simulink model "SelfBalancingEV_V2"  (R2022a)
settings: Solver=VariableStepAuto  StartTime=0.0  StopTime=30  RelTol=1e-3
undefined symbols (not defined in the file): Ion, Lithium, sigbuilder_block, X, Y, Z
libraries: sm_lib x26, simulink x8, nesl_utility x6, fl_lib x3, slpidlib x2, spsControlledCurrentSourceLib x1, spsBatteryLib x1, spspowerguiLib x1
(part 1 of 2)
settings Model: Creator=DELL  LastModifiedBy=DELL
settings ConfigComp: CovScope=ReferencedModels

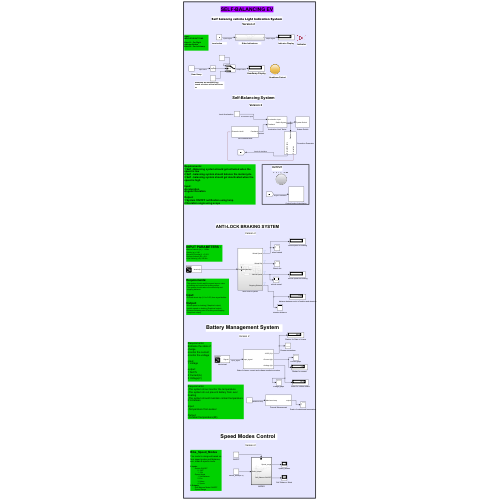
[thumbnail: Simulink's stored preview of the top-level diagram]
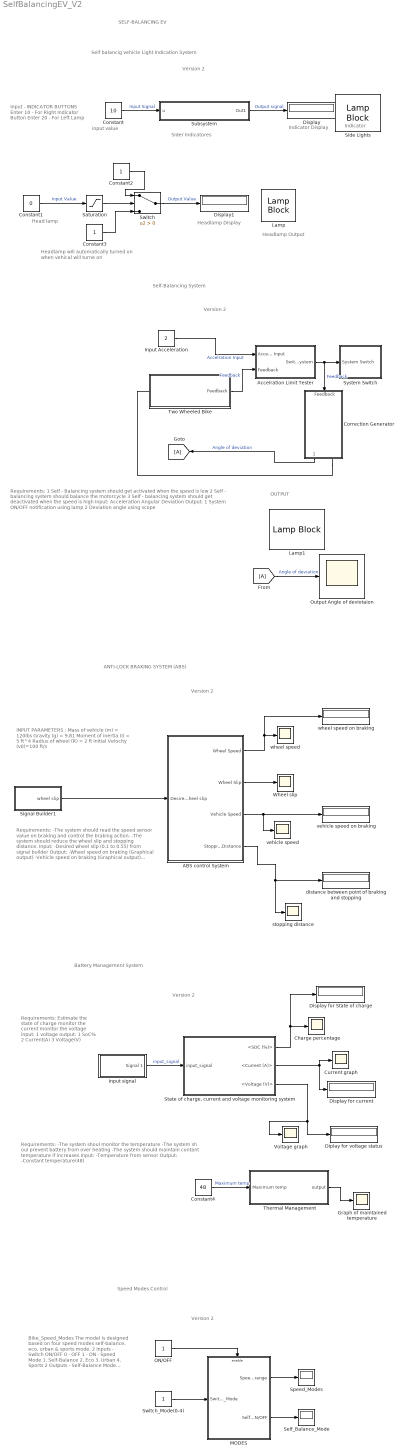
== system SelfBalancingEV_V2 ==
  note: SELF-BALANCING EV
  note: input value
  note: Head lamp
  note: Indicator Display
  note: Input -
      | INDICATOR BUTTONS
      |
      | Enter 10 - For Right Indicator Button
      | Enter 20 - For Left Lamp
  note: Indicator
  note: Version 2
  note: Headlamp Display
  note: Self balancig vehicle Light Indication System
  note: Headlamp will automatically turned on when vehical will turne on
  note: Sider Indicatores
  note: Headlamp Output
  note: Requirements:
      | -The system should read the speed sensor value
      | on braking and control the braking action.
      | -The system should reduce the wheel slip and
      | stopping distance.
      |
      | Input:
      | -Desired wheel slip (0.1 to 0.55) from signal builder
      |
      | Output:
      | -Wheel speed on braking (Graphical output)
      | -Vehicle speed on braking (Graphical output)
      | -Distance between point of braking and stopping
      | (Graphical output)
  note: INPUT PARAMETERS :
      | Mass of vehicle (m) = 120lbs
      | Gravity (g) = 9.81
      | Moment of inertia (I) = 5 ft^4
      | Radius of wheel (R) = 2 ft
      | Initial Velocity (v0)=100 ft/s
  note: ANTI-LOCK BRAKING SYSTEM (ABS)
  note: Version 2
  note: Requirements:
      | -The system shoul monitor the temperature
      | -The system sh oul prevent battery from over
      | heating
      | -The system should maintain contant temperature
      | if increases
      |
      | Input:
      | -Temperature from sensor
      |
      | Output:
      | -Constant temperature(48)
  note: Battery Management System
  note: Requirements:
      | Estimate the state of
      | charge
      | monitor the current
      | monitor the voltage
      |
      | input:
      | 1 voltage
      |
      | output:
      | 1 SoC%
      | 2 Current(A)
      | 3 Voltage(V)
  note: Bike_Speed_Modes
      |
      | The model is designed based on
      | four speed modes self-balance,
      | eco, urban & sports mode.
      |
      | 2 Inputs
      | - Switch ON/OFF
      | 0 - OFF
      | 1 - ON
      | - Speed Mode
      | 1. Self-Balance
      | 2. Eco
      | 3. Urban
      | 4. Sports
      | 2 Outputs
      | - Self-Balance Mode ON/OFF
      | - Speed Range
  note: Version 2
  note: Speed Modes Control
  note: Version 2
  note: Requirements:
      | 1 Self - Balancing system should get activated when the speed is low
      | 2 Self - balancing system should balance the motorcycle
      | 3 Self - balancing system should get deactivated when the speed is high
      |
      | Input:
      | Acceleration
      | Angular Deviation
      |
      | Output:
      | 1 System ON/OFF notification using lamp
      | 2 Deviation angle using scope
  note: Self-Balancing System
  note: OUTPUT
  note: Version 2
  ABS control System : Subsystem
  Accelration Limit Tester : Subsystem
  Charge percentage : Scope
  Constant : Constant  Value=10
  Constant1 : Constant  Value=0
  Constant2 : Constant
  Constant3 : Constant
  Constant4 : Constant  Value=48
  Correction Generator : Subsystem
  Current graph : Scope
  Diplay for voltage status : Display
  Display : Display
  Display for State of charge : Display
  Display for current : Display
  Display1 : Display
  From : From
  Goto : Goto
  Graph of maintained temperature : Scope
  Input Acceleration : Constant  Value=2
  Input signal : Subsystem  Tag=STV Subsys  LoadFcn=sigbuilder_block('load');  StartFcn=sigbuilder_block('start');  StopFcn=sigbuilder_block('stop');  ClipboardFcn=sigbuilder_block('clipboard');  mask(Sigbuilder block){tuvar=[0:10]}
      mask help: Simulink:masks:SigbuilderBlock_MD
      mask init:
      | if ~strcmp(get_param(bdroot(gcbh),'SimulationStatus'),'stopped') tuvar = sigbuilder_block('maskInit'); end
      settings: CopyFcn=sigbuilder_block('copy');  DeleteFcn=sigbuilder_block('delete');  ModelCloseFcn=sigbuilder_block('modelClose');  PreSaveFcn=sigbuilder_block('preSave');  PauseFcn=sigbuilder_block('pause');  ContinueFcn=sigbuilder_block('continue');  NameChangeFcn=sigbuilder_block('namechange');  OpenFcn=sigbuilder_block('open',[406.8 120.6 550.8 400.2 ]);  CloseFcn=sigbuilder_block('close');
      mask Display: plot(0, 0, 100, 100,[2, 2, 32, 32, 2], [68, 8, 8, 68, 68],[32, 2], [38, 38], [32, 19, 2],[53, 60, 44], [32, 17, 17, 2],[16, 16, 31, 31]);txt = getActiveGroup(gcbh);text(2, 100, txt,'verticalAlignment', 'top');
  Lamp : LampBlock  LabelPosition=Hide
  Lamp1 : LampBlock
  MODES : Subsystem
  ON/OFF : Constant
  "Output Angle of deviotaion " : Scope
  Saturation : Saturate  UpperLimit=1  LowerLimit=0
  Self_Balance_Mode : Display
  Side Lights : LampBlock  LabelPosition=Hide  Icon=SideLights
  Signal Builder1 : Subsystem  Tag=STV Subsys  LoadFcn=sigbuilder_block('load');  StartFcn=sigbuilder_block('start');  StopFcn=sigbuilder_block('stop');  ClipboardFcn=sigbuilder_block('clipboard');  mask(Sigbuilder block){tuvar=[0:10]}
      mask help: Simulink:masks:SigbuilderBlock_MD
      mask init:
      | if ~strcmp(get_param(bdroot(gcbh),'SimulationStatus'),'stopped') tuvar = sigbuilder_block('maskInit'); end
      settings: CopyFcn=sigbuilder_block('copy');  DeleteFcn=sigbuilder_block('delete');  ModelCloseFcn=sigbuilder_block('modelClose');  PreSaveFcn=sigbuilder_block('preSave');  PauseFcn=sigbuilder_block('pause');  ContinueFcn=sigbuilder_block('continue');  NameChangeFcn=sigbuilder_block('namechange');  OpenFcn=sigbuilder_block('open',[437.6 199.2 550.4 400 ]);  CloseFcn=sigbuilder_block('close');
      mask Display: plot(0, 0, 100, 100,[2, 2, 32, 32, 2], [68, 8, 8, 68, 68],[32, 2], [38, 38], [32, 19, 2],[53, 60, 44], [32, 17, 17, 2],[16, 16, 31, 31]);txt = getActiveGroup(gcbh);text(2, 100, txt,'verticalAlignment', 'top');
  Speed_Modes : Display
  "State of charge, current and voltage monitoring system" : Subsystem
  Subsystem : Subsystem
  Switch : Switch  Criteria=u2 > Threshold  SaturateOnIntegerOverflow=off  InputSameDT=off
  Switch_Mode(0-4) : Constant
  System Switch : Subsystem
  Thermal Management : Subsystem
  Two Wheeled Bike : Subsystem
  "Voltage graph " : Scope
  Wheel slip : Scope
  distance between point of braking and stopping : Display
  stopping distance : Scope
  vehicle speed : Scope
  vehicle speed on braking : Display
  wheel speed : Scope
  wheel speed on braking : Display
  wires:
  Constant1/1 -> Saturation/1  "Input Value"
  Subsystem/1(Out1) -> Display/1  "Output signal"
  Saturation/1 -> Switch/2
  Switch/1 -> Display1/1  "Output Value"
  Constant/1 -> Subsystem/1(u)  "Input Signal"
  Constant2/1 -> Switch/1
  Constant3/1 -> Switch/3
  ABS control System/4(Stopping Distance) -> distance between point of braking and stopping/1, stopping distance/1
  ABS control System/1(Wheel Speed) -> wheel speed/1, wheel speed on braking/1
  ABS control System/2(Wheel Slip) -> Wheel slip/1
  ABS control System/3(Vehicle Speed) -> vehicle speed on braking/1, vehicle speed/1
  Signal Builder1/1(wheel slip) -> ABS control System/1(Desired wheel slip)
  Constant4/1 -> Thermal Management/1(Maximum temp)  "Maximum temp"
  Input signal/1(Signal 1) -> "State of charge, current and voltage monitoring system"/1(input_signal)  "input_signal"
  "State of charge, current and voltage monitoring system"/1(<SOC (%)>) -> Display for State of charge/1, Charge percentage/1
  Thermal Management/1(output) -> Graph of maintained temperature/1
  "State of charge, current and voltage monitoring system"/2(<Current (A)>) -> Current graph/1, Display for current/1
  "State of charge, current and voltage monitoring system"/3(<Voltage (V)>) -> Diplay for voltage status/1, "Voltage graph "/1
  MODES/1(Speed_range) -> Speed_Modes/1
  MODES/2(Self_Balance ON/OFF) -> Self_Balance_Mode/1
  Switch_Mode(0-4)/1 -> MODES/1(Swithc_Mode)
  ON/OFF/1 -> MODES/Enable
  From/1 -> "Output Angle of deviotaion "/1  "Angle of deviation"
  Correction Generator/1(Deviation Angle) -> Goto/1  "Angle of deviation"
  Input Acceleration/1 -> Accelration Limit Tester/1(Acceleration Input)  "Accelration Input"
  Two Wheeled Bike/1(Feedback) -> Accelration Limit Tester/2("Feedback ")  "Feedback"
  Accelration Limit Tester/1(Switch System) -> System Switch/1(System Switch), Correction Generator/1(Feedback)  "Feedback"
  connections:
  Correction Generator/RConn1 -- Two Wheeled Bike/LConn1

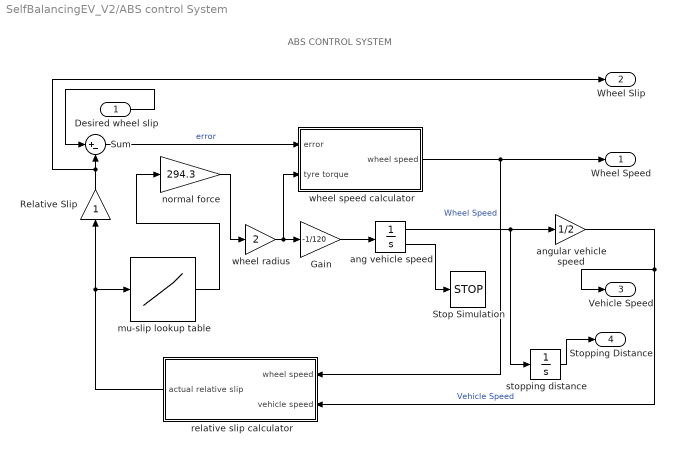
== system SelfBalancingEV_V2/ABS control System ==
  note: ABS CONTROL SYSTEM
  Desired wheel slip : Inport
  Gain : Gain  Gain=-1/120
  Relative Slip : Gain
  Stop Simulation : Stop
  Sum : Sum  Inputs=|+-
  ang vehicle speed : Integrator  InitialCondition=100  LimitOutput=on  UpperSaturationLimit=1000  LowerSaturationLimit=0  ShowSaturationPort=on
  angular vehicle speed : Gain  Gain=1/2
  mu-slip lookup table : Lookup_n-D  NumberOfTableDimensions=1  BreakpointsForDimension1=[0;0.05;0.1;0.15;0.2;0.25;0.3;0.35;0.4;0.45;0.5;0.55;0.6;0.65;0.7;0.75;0.8;0.85;0.9;0.95;1]  Table=[0;0.4;0.8;0.97;1;0.98;0.96;0.94;0.92;0.9;0.88;0.855;0.83;0.81;0.79;0.77;0.75;0.73;0.72;0.71;0.7]  InternalRulePriority=Speed  RndMeth=Simplest
  normal force : Gain  Gain=294.3
  relative slip calculator : Subsystem
  stopping distance : Integrator
  wheel radius : Gain  Gain=2
  wheel speed calculator : Subsystem
  Wheel Speed : Outport
  Wheel Slip : Outport  Port=2
  Vehicle Speed : Outport  Port=3
  Stopping Distance : Outport  Port=4
  wires:
  ang vehicle speed/1 -> angular vehicle speed/1, stopping distance/1
  relative slip calculator/1(actual relative slip) -> Relative Slip/1, mu-slip lookup table/1
  normal force/1 -> wheel radius/1
  wheel speed calculator/1(wheel speed) -> Wheel Speed/1, relative slip calculator/1(wheel speed)  "Wheel Speed"
  Sum/1 -> wheel speed calculator/1(error)  "error"
  angular vehicle speed/1 -> Vehicle Speed/1, relative slip calculator/2(vehicle speed)  "Vehicle Speed"
  Gain/1 -> ang vehicle speed/1
  wheel radius/1 -> Gain/1, wheel speed calculator/2(tyre torque)
  ang vehicle speed/2 -> Stop Simulation/1
  Relative Slip/1 -> Wheel Slip/1, Sum/2
  mu-slip lookup table/1 -> normal force/1
  stopping distance/1 -> Stopping Distance/1
  Desired wheel slip/1 -> Sum/1

== system SelfBalancingEV_V2/Accelration Limit Tester ==
  note: Requirement
      | 1 Acceleration tester which enables the system at low speed
      |
      | Input
      | 1 Acceleration
      |
      | Output
      | 1 Feedback
  note: Accelration Limit Tester
  Acceleration Input : Inport
  "Feedback " : Inport  Port=2
  Switch1 : Switch  Threshold=4  SaturateOnIntegerOverflow=off  InputSameDT=off
  const : Constant  Value=0
  Switch System : Outport
  wires:
  Acceleration Input/1 -> Switch1/2  "Acceleration Input"
  const/1 -> Switch1/1
  "Feedback "/1 -> Switch1/3  "Feedback"
  Switch1/1 -> Switch System/1  "Feedback"

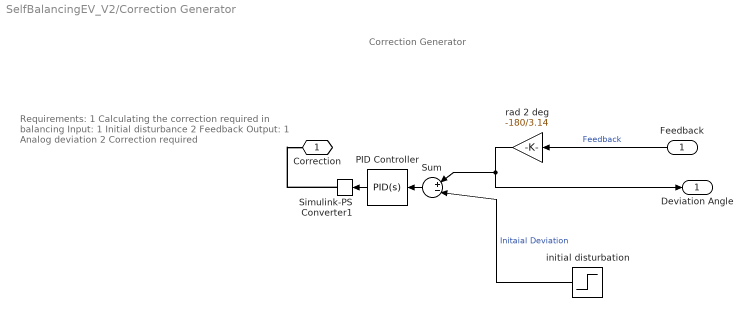
== system SelfBalancingEV_V2/Correction Generator ==
  note: Requirements:
      | 1 Calculating the correction required in balancing
      | Input:
      | 1 Initial disturbance
      | 2 Feedback
      |
      | Output:
      | 1 Analog deviation
      | 2 Correction required
  note: Correction Generator
  Feedback : Inport
  PID Controller : slpidlib/PID Controller  Controller=PID  Form=Parallel  TimeDomain=Continuous-time  UseExternalTs=off  SampleTime=-1  IntegratorMethod=Forward Euler  FilterMethod=Forward Euler  ControllerParametersSource=internal  P=2  I=5  UseKiTs=off  D=0.01  N=100  UseFilter=on  TunerSelectOption=Transfer Function Based (PID Tuner App)  InitialConditionSource=internal  InitialConditionForIntegrator=0  InitialConditionForFilter=0  DifferentiatorICPrevScaledInput=0  ExternalReset=none  TrackingMode=off  Kt=1  LimitOutput=off  SatLimitsSource=internal  UpperSaturationLimit=inf  LowerSaturationLimit=-inf  LinearizeAsGain=on  AntiWindupMode=none  Kb=1  POutMin=[]  POutMax=[]  IOutMin=[]  IOutMax=[]  DOutMin=[]  DOutMax=[]  NOutMin=[]  NOutMax=[]  SumOutMin=[]  SumOutMax=[]  SaturationOutMin=[]  SaturationOutMax=[]  PParamMin=[]  PParamMax=[]  IParamMin=[]  IParamMax=[]  DParamMin=[]  DParamMax=[]  NParamMin=[]  NParamMax=[]  KbParamMin=[]  KbParamMax=[]  KtParamMin=[]  KtParamMax=[]  KbOutMin=[]  KbOutMax=[]  KtOutMin=[]  KtOutMax=[]  IntegratorOutMin=[]  IntegratorOutMax=[]  FilterOutMin=[]  FilterOutMax=[]  SumI1OutMin=[]  SumI1OutMax=[]  SumI2OutMin=[]  SumI2OutMax=[]  SumI3OutMin=[]  SumI3OutMax=[]  SumI4OutMin=[]  SumI4OutMax=[]  SumDOutMin=[]  SumDOutMax=[]  DifferentiatorOutMin=[]  DifferentiatorOutMax=[]  FilterDiffOutCoefMin=[]  FilterDiffOutCoefMax=[]  ReciprocalOutMin=[]  ReciprocalOutMax=[]  SumDenOutMin=[]  SumDenOutMax=[]  SumNumOutMin=[]  SumNumOutMax=[]  DivideOutMin=[]  DivideOutMax=[]  UdiffTsProdOutMin=[]  UdiffTsProdOutMax=[]  NTsProdOutMin=[]  NTsProdOutMax=[]  UintegralTsProdOutMin=[]  UintegralTsProdOutMax=[]  UngainTsProdOutMin=[]  UngainTsProdOutMax=[]  IntegratorContinuousStateAttributes=''  IntegratorStateMustResolveToSignalObject=off  IntegratorRTWStateStorageClass=Auto  FilterContinuousStateAttributes=''  FilterStateMustResolveToSignalObject=off  FilterRTWStateStorageClass=Auto  ParallelPVariant=InternalParameters  IdealPVariant=Disabled  IVariant=InternalParameters  DVariant=InternalParameters  IntegratorVariant=Continuous  SatVariant=Disabled  AWVariant=Passthrough  PCopyVariant=Disabled  TRVariant=Disabled  FdbkBlocksVariant=Forward  IdealPFdbkVariant=Disabled  SatFdbkVariant=Disabled  DerivativeFilterVariant=ContFilter  NVariant=InternalParameters  NCopyVariant=Disabled  FilterICVariant=InternalICsFilter  IntegratorICVariant=InternalICs  ExternalResetVariant=Disabled  TRSumVariant=Passthrough  SumFdbkVariant=Disabled  SumVariant=Sum_PID  TsampFilterVariant=InternalTs  TsampNgainVariant=Passthrough  TsampIntegralVariant=Passthrough  ExternalSaturationOutDataTypeStr=Inherit: Same as second input  aMode=0
  Simulink-PS Converter1 : nesl_utility/Simulink-PS Converter  PhysicalDomain=network_engine_domain  SubClassName=ps_input  LeftPortType=input  RightPortType=output  PseudoPeriodic=off  Frequencies=[]  NoiseDistribution=none  NoiseParameters=[]  Unit=N  AffineConversion=off  FilteringAndDerivatives=filter  SimscapeFilterOrder=2  InputFilterTimeConstant=0.001  UdotUserProvided=0
  Sum : Sum  Inputs=|+-|
  initial disturbation : Step  Time=0.01  Before=10  After=0  SampleTime=0
  rad 2 deg : Gain  Gain=-180/3.14
  Correction : PMIOPort  Side=Right
  Deviation Angle : Outport
  wires:
  rad 2 deg/1 -> Deviation Angle/1, Sum/1
  Sum/1 -> PID Controller/1
  Feedback/1 -> rad 2 deg/1  "Feedback"
  PID Controller/1 -> Simulink-PS Converter1/1
  initial disturbation/1 -> Sum/2  "Initaial Deviation"
  connections:
  Simulink-PS Converter1/RConn1 -- Correction/RConn1

== system SelfBalancingEV_V2/Input signal ==
  Demux : Demux  Tag=STV Demux  Outputs=1
      settings: DisplayOption=none
  FromWs : FromWorkspace  Tag=STV FromWs  VariableName=tuvar
      SigBuilderData=|
      | common.afterFinalStr = 'Extrapolate'
      | common.sampleTime = 0
      | dataSet.timeRange = [0 10]
      | dataSet.name = 'Group 1'
      | sbobj.Groups.Name = 'Group 1'
      | sbobj.Groups.Signals.Name = 'Signal 1'
      | sbobj.Groups.Signals.XData = [0 1.94 2.9 4 4 4.88 5.44 5.98 6.66 6.66 7.76 10]
      | sbobj.Groups.Signals.YData = [0 0.62 0.485 0 0.82 0.875 0.255 0.005 1 0 0.42 0]
  Signal 1 : Outport  Tag=STV Outport
  wires:
  Demux/1 -> Signal 1/1
  FromWs/1 -> Demux/1

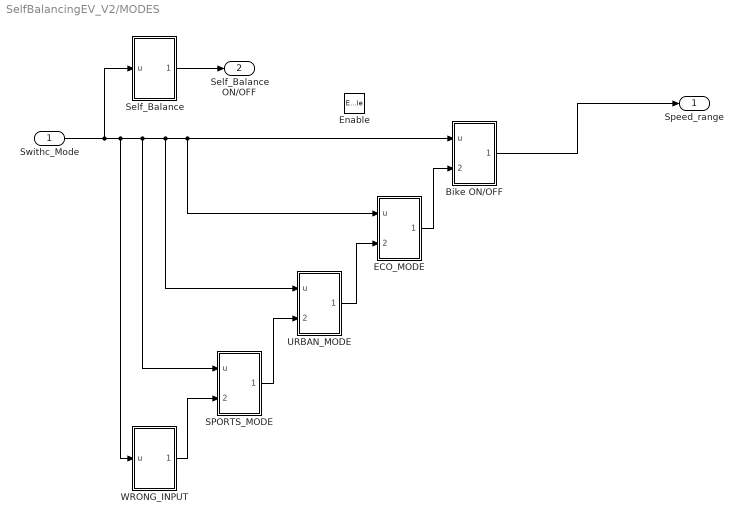
== system SelfBalancingEV_V2/MODES ==
  Swithc_Mode : Inport
  Enable : EnablePort
  Bike ON/OFF : Subsystem
  ECO_MODE : Subsystem
  SPORTS_MODE : Subsystem
  Self_Balance : Subsystem
  URBAN_MODE : Subsystem
  WRONG_INPUT : Subsystem
  Speed_range : Outport
  Self_Balance ON/OFF : Outport  Port=2
  wires:
  Swithc_Mode/1 -> Bike ON/OFF/1(u), ECO_MODE/1(u), URBAN_MODE/1(u), SPORTS_MODE/1(u), WRONG_INPUT/1(u), Self_Balance/1(u)
  Self_Balance/1(Out1) -> Self_Balance ON/OFF/1
  Bike ON/OFF/1(Out1) -> Speed_range/1
  ECO_MODE/1(Out1) -> Bike ON/OFF/2(In2)
  URBAN_MODE/1(Out1) -> ECO_MODE/2(In2)
  SPORTS_MODE/1(Out1) -> URBAN_MODE/2(In2)
  WRONG_INPUT/1(Out1) -> SPORTS_MODE/2(In2)

== system SelfBalancingEV_V2/Signal Builder1 ==
  Demux : Demux  Tag=STV Demux  Outputs=1
      settings: DisplayOption=none
  FromWs : FromWorkspace  Tag=STV FromWs  VariableName=tuvar
      SigBuilderData=|
      | common.afterFinalStr = 'Extrapolate'
      | common.sampleTime = 0
      | dataSet.timeRange = [1 10]
      | dataSet.name = 'Sheet1'
      | sbobj.Groups.Name = 'Sheet1'
      | sbobj.Groups.Signals.Name = 'wheel slip'
      | sbobj.Groups.Signals.XData = [1 2 3 4 5 6 7 8 9 10]
      | sbobj.Groups.Signals.YData = [0.1 0.15 0.2 0.25 0.3 0.35 0.4 0.45 0.5 0.55]
      | sbobj.Groups.TimeRange = [1 10]
  wheel slip : Outport  Tag=STV Outport
  wires:
  Demux/1 -> wheel slip/1
  FromWs/1 -> Demux/1

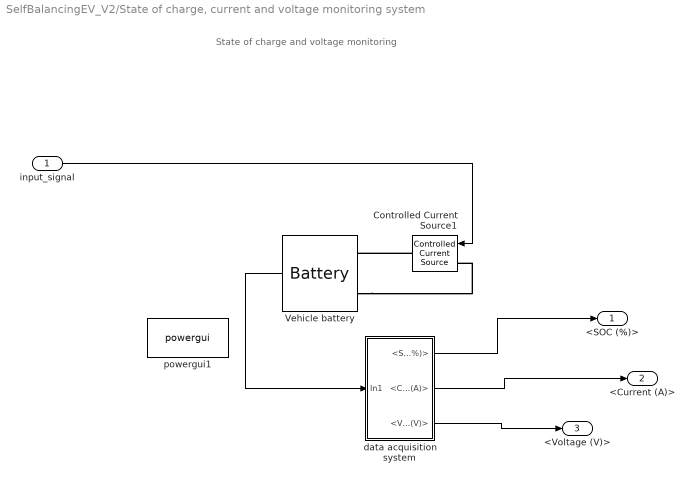
== system SelfBalancingEV_V2/State of charge, current and voltage monitoring system ==
  note: State of charge and voltage monitoring
  input_signal : Inport
  Controlled Current Source1 : spsControlledCurrentSourceLib/Controlled Current Source  Initialize=on  Source_Type=AC  Amplitude=0  Phase=0  Frequency=0  Measurements=None
  Vehicle battery : spsBatteryLib/Battery  BatType=Lithium-Ion  ShowTempParam=off  ThermalPreset=no  ShowAgeParam=off  NomV=50  NomQ=50  SOC=100  Batt_Tr=30  PresetModel=on  MaxQ=50  MinV=37.5  FullV=58.1994  Dis_rate=21.7391  R=0.01  Normal_OP=45.2174  expZone="[54.0193      2.45652]"  current=[6.5 13 32.5]  Units=Time  Tci=20  NomT=20  T2=-30  MaxQ2=4.8  FullV2=7.1  Normal_OP2=5.655  expZone2="[6.58           1]"  Rca=0.6  ti=2000  Dp=0  Neq0=0  Tsim=1e6  Ta1=25  Qeol=5.4*0.9  Reol=0.013333*1.2  Char_age=[2.3478, 3]  Dis_age=[2.3478, 10]  N1=1500  N2=10500  N3=1000  N4=1400  Ta2=45  N5=950
  data acquisition system : Subsystem
  powergui1 : spspowerguiLib/powergui  Priority=1  SimulationMode=Continuous  SampleTime=50e-6  frequency=60  Iterations=50  frequencyindice=0  Pbase=100e6  ErrMax=1e-4  UnitsV=kV  UnitsW=MW  buscounter=0  FunctionMessages=off  echomessages=off  EnableUseOfTLC=off  CurrentSourceSwitches=off  DisableSnubberDevices=off  DisableRonSwitches=off  DisableVfSwitches=off  DisplayEquations=off  AutomaticDiscreteSolvers=off  SolverType=Tustin/Backward Euler (TBE)  Interpol=off  ExternalGateDelay=off  methode=off  Ts=100  x0status=blocks  SPID=on  SwTol=0  HookPort=off  NonlinearTolerance=1e-4  nMaxIteration=100  ContinueOnMaxIteration=off  RestoreLinks=warning  ResistiveCurrentMeasurement=off  Frange=[0:2:500]  Ylog=off  Xlog=on  ShowGrid=off  save=off  variable=ZData  structure=0  ZoomFFT=off  StartTime=0.0  cycles=1  DisplayStyle=1  fundamental=60  FreqAxis=off  MaxFrequency=1000  frequencyindicesteady=1  RmsSteady=1  display=off
  <SOC (%)> : Outport
  <Current (A)> : Outport  Port=2
  <Voltage (V)> : Outport  Port=3
  wires:
  input_signal/1 -> Controlled Current Source1/1
  Vehicle battery/1 -> data acquisition system/1(In1)
  data acquisition system/1(<SOC (%)>) -> <SOC (%)>/1
  data acquisition system/2(<Current (A)>) -> <Current (A)>/1
  data acquisition system/3(<Voltage (V)>) -> <Voltage (V)>/1
  connections:
  Controlled Current Source1/RConn1 -- Vehicle battery/LConn1
  Vehicle battery/LConn2 -- Controlled Current Source1/LConn1

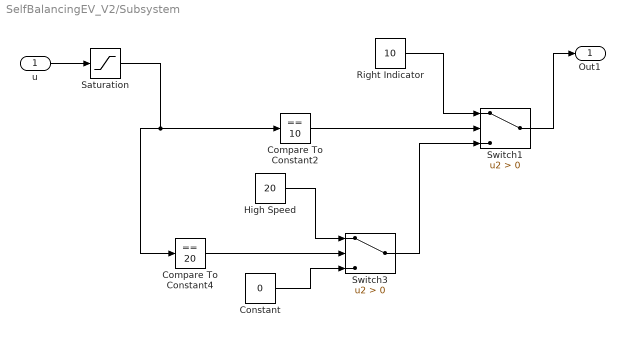
== system SelfBalancingEV_V2/Subsystem ==
  u : Inport
  Compare To Constant2 : simulink/Logic and Bit Operations/Compare To Constant  relop===  const=10  OutDataTypeStr=boolean
  Compare To Constant4 : simulink/Logic and Bit Operations/Compare To Constant  relop===  const=20  OutDataTypeStr=boolean
  Constant : Constant  Value=0
  High Speed : Constant  Value=20
  Right Indicator : Constant  Value=10
  Saturation : Saturate  UpperLimit=20  LowerLimit=0
  Switch1 : Switch  Criteria=u2 > Threshold  SaturateOnIntegerOverflow=off  InputSameDT=off
  Switch3 : Switch  Criteria=u2 > Threshold  SaturateOnIntegerOverflow=off  InputSameDT=off
  Out1 : Outport
  wires:
  Compare To Constant2/1 -> Switch1/2
  u/1 -> Saturation/1
  Compare To Constant4/1 -> Switch3/2
  Switch3/1 -> Switch1/3
  Right Indicator/1 -> Switch1/1
  High Speed/1 -> Switch3/1
  Constant/1 -> Switch3/3
  Switch1/1 -> Out1/1
  Saturation/1 -> Compare To Constant4/1, Compare To Constant2/1

== system SelfBalancingEV_V2/System Switch ==
  note: Requirements:
      | 1 Displaying the system state
      |
      | Input:
      | 1 Feedback
      |
      | Output
      | 1 System state
  note: System Switch
  System Switch : Inport
  Constant : Constant
  Constant1 : Constant  Value=0
  Display : Display
  System Status ON/OFF : Switch  Criteria=u2 ~= 0  SaturateOnIntegerOverflow=off  InputSameDT=off
  wires:
  Constant1/1 -> System Status ON/OFF/3
  System Switch/1 -> System Status ON/OFF/2
  Constant/1 -> System Status ON/OFF/1
  System Status ON/OFF/1 -> Display/1

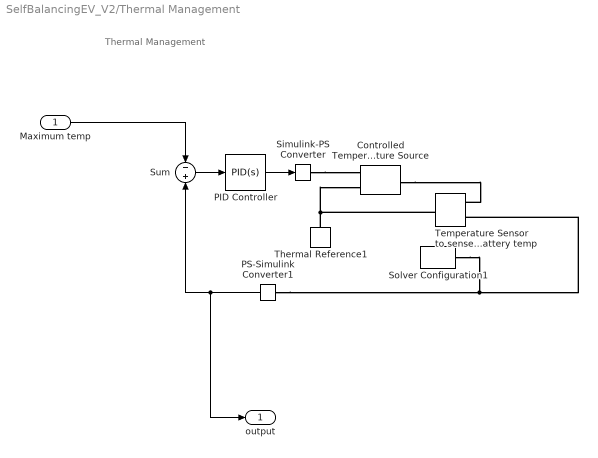
== system SelfBalancingEV_V2/Thermal Management ==
  note: Thermal Management
  Maximum temp : Inport
  Controlled Temperature Source : fl_lib/Thermal/Thermal Sources/Controlled Temperature Source
  PID Controller : slpidlib/PID Controller  Controller=PID  Form=Parallel  TimeDomain=Continuous-time  UseExternalTs=off  SampleTime=-1  IntegratorMethod=Forward Euler  FilterMethod=Forward Euler  ControllerParametersSource=internal  P=1  I=1  UseKiTs=off  D=0  N=100  UseFilter=on  TunerSelectOption=Transfer Function Based (PID Tuner App)  InitialConditionSource=internal  InitialConditionForIntegrator=0  InitialConditionForFilter=0  DifferentiatorICPrevScaledInput=0  ExternalReset=none  TrackingMode=off  Kt=1  LimitOutput=off  SatLimitsSource=internal  UpperSaturationLimit=inf  LowerSaturationLimit=-inf  LinearizeAsGain=on  AntiWindupMode=none  Kb=1  POutMin=[]  POutMax=[]  IOutMin=[]  IOutMax=[]  DOutMin=[]  DOutMax=[]  NOutMin=[]  NOutMax=[]  SumOutMin=[]  SumOutMax=[]  SaturationOutMin=[]  SaturationOutMax=[]  PParamMin=[]  PParamMax=[]  IParamMin=[]  IParamMax=[]  DParamMin=[]  DParamMax=[]  NParamMin=[]  NParamMax=[]  KbParamMin=[]  KbParamMax=[]  KtParamMin=[]  KtParamMax=[]  KbOutMin=[]  KbOutMax=[]  KtOutMin=[]  KtOutMax=[]  IntegratorOutMin=[]  IntegratorOutMax=[]  FilterOutMin=[]  FilterOutMax=[]  SumI1OutMin=[]  SumI1OutMax=[]  SumI2OutMin=[]  SumI2OutMax=[]  SumI3OutMin=[]  SumI3OutMax=[]  SumI4OutMin=[]  SumI4OutMax=[]  SumDOutMin=[]  SumDOutMax=[]  DifferentiatorOutMin=[]  DifferentiatorOutMax=[]  FilterDiffOutCoefMin=[]  FilterDiffOutCoefMax=[]  ReciprocalOutMin=[]  ReciprocalOutMax=[]  SumDenOutMin=[]  SumDenOutMax=[]  SumNumOutMin=[]  SumNumOutMax=[]  DivideOutMin=[]  DivideOutMax=[]  UdiffTsProdOutMin=[]  UdiffTsProdOutMax=[]  NTsProdOutMin=[]  NTsProdOutMax=[]  UintegralTsProdOutMin=[]  UintegralTsProdOutMax=[]  UngainTsProdOutMin=[]  UngainTsProdOutMax=[]  IntegratorContinuousStateAttributes=''  IntegratorStateMustResolveToSignalObject=off  IntegratorRTWStateStorageClass=Auto  FilterContinuousStateAttributes=''  FilterStateMustResolveToSignalObject=off  FilterRTWStateStorageClass=Auto  ParallelPVariant=InternalParameters  IdealPVariant=Disabled  IVariant=InternalParameters  DVariant=InternalParameters  IntegratorVariant=Continuous  SatVariant=Disabled  AWVariant=Passthrough  PCopyVariant=Disabled  TRVariant=Disabled  FdbkBlocksVariant=Forward  IdealPFdbkVariant=Disabled  SatFdbkVariant=Disabled  DerivativeFilterVariant=ContFilter  NVariant=InternalParameters  NCopyVariant=Disabled  FilterICVariant=InternalICsFilter  IntegratorICVariant=InternalICs  ExternalResetVariant=Disabled  TRSumVariant=Passthrough  SumFdbkVariant=Disabled  SumVariant=Sum_PID  TsampFilterVariant=InternalTs  TsampNgainVariant=Passthrough  TsampIntegralVariant=Passthrough  ExternalSaturationOutDataTypeStr=Inherit: Same as second input  aMode=0
  PS-Simulink Converter1 : nesl_utility/PS-Simulink Converter  PhysicalDomain=network_engine_domain  SubClassName=ps_output  LeftPortType=input  RightPortType=output  PseudoPeriodic=off  Frequencies=[]  VectorFormat=1-D array  Unit=inherit  AffineConversion=off
  Simulink-PS Converter : nesl_utility/Simulink-PS Converter  PhysicalDomain=network_engine_domain  SubClassName=ps_input  LeftPortType=input  RightPortType=output  PseudoPeriodic=off  Frequencies=[]  NoiseDistribution=none  NoiseParameters=[]  Unit=1  AffineConversion=off  FilteringAndDerivatives=provide  SimscapeFilterOrder=1  InputFilterTimeConstant=0.001  UdotUserProvided=0
  Solver Configuration1 : nesl_utility/Solver Configuration  PhysicalDomain=network_engine_domain  SubClassName=solver  LeftPortType=input  RightPortType=generic  Tones=[]  Harmonics=[]  SimulateNoise=off  Profile=off  UseLocalSampling=off  EnableSwitchedLinearOptims=on  FrequencyDomain=off  UseCCode=off  RelTol=0.001  AbsTol=1e-06  MinStep=1e-09  ToWorkspace=off  RevertToSquareIcSolve=off  NumHomotopyIterations=100  PhasorMode=off  PhasorModeNumHarmonics=1  IndexReductionMethod=DerivativeReplacement  DoDC=off  ResidualTolerance=1e-09  UseLocalSolver=off  LocalSolverChoice=NE_BACKWARD_EULER_ADVANCER  LocalSolverSampleTime=0.001  DoFixedCost=off  MaxNonlinIter=3  MaxModeIter=2  ComputeImpulses=off  ImpulseIterations=2  LinearAlgebra=auto  LinearAlgebraNumThread=0  EquationFormulation=NE_TIME_EF  DelaysMemoryBudget=1024  AutomaticFiltering=on  FilteringTimeConstant=0.001  PartitionStorageMethod=AS_NEEDED  PartitionMemoryBudget=1024  PartitionMethod=ROBUST
  Sum : Sum  Inputs=-+
  Temperature Sensor to sense the battery temp : fl_lib/Thermal/Thermal Sensors/Temperature Sensor
  Thermal Reference1 : fl_lib/Thermal/Thermal Elements/Thermal Reference
  output : Outport
  wires:
  PS-Simulink Converter1/1 -> output/1, Sum/2
  PID Controller/1 -> Simulink-PS Converter/1
  Maximum temp/1 -> Sum/1
  Sum/1 -> PID Controller/1
  connections:
  Controlled Temperature Source/LConn1 -- Temperature Sensor to sense the battery temp/RConn1
  Thermal Reference1/LConn1 -- Temperature Sensor to sense the battery temp/LConn1 -- Controlled Temperature Source/RConn2
  Simulink-PS Converter/RConn1 -- Controlled Temperature Source/RConn1
  PS-Simulink Converter1/LConn1 -- Solver Configuration1/RConn1 -- Temperature Sensor to sense the battery temp/RConn2

== system SelfBalancingEV_V2/Two Wheeled Bike ==
  note: Requirements:
      | 1 Building the physical model for calculationg the result and momentum
      |
      | Output:
      | 1 Feedback
      |
      | Input:
      | 1 World frame
  note: Two wheeled Bike
  Momenturm Calculation Block : Subsystem
  Physical Block : Subsystem
  World Frame : Subsystem
  Prismatic Joint2 : PMIOPort  Side=Left
  Feedback : Outport
  wires:
  Momenturm Calculation Block/1(output) -> Feedback/1  "Feedback"
  connections:
  Physical Block/LConn2 -- Momenturm Calculation Block/RConn2
  Momenturm Calculation Block/LConn1 -- World Frame/RConn1
  Prismatic Joint2/RConn1 -- Momenturm Calculation Block/LConn2
  Physical Block/LConn1 -- Momenturm Calculation Block/RConn1

== system SelfBalancingEV_V2/ABS control System/relative slip calculator ==
  note: Relative Slip Calculater
  wheel speed : Inport
  vehicle speed : Inport  Port=2
  Constant : Constant
  Divide : Product  Inputs=*/
  Sum1 : Sum  Inputs=|+-
  actual relative slip : Outport
  wires:
  Divide/1 -> Sum1/2
  vehicle speed/1 -> Divide/2
  wheel speed/1 -> Divide/1
  Sum1/1 -> actual relative slip/1  "actual relative slip"
  Constant/1 -> Sum1/1

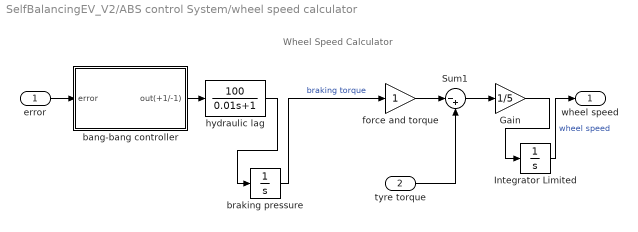
== system SelfBalancingEV_V2/ABS control System/wheel speed calculator ==
  note: Wheel Speed Calculator
  error : Inport
  tyre torque : Inport  Port=2
  Gain : Gain  Gain=1/5
  Integrator Limited : Integrator  InitialCondition=100/2  LimitOutput=on  UpperSaturationLimit=1000  LowerSaturationLimit=0
  Sum1 : Sum  Inputs=|-+
  bang-bang controller : Subsystem
  braking pressure : Integrator  LimitOutput=on  UpperSaturationLimit=1000  LowerSaturationLimit=0
  force and torque : Gain
  hydraulic lag : TransferFcn  Numerator=[100]  Denominator=[0.01 1]
  wheel speed : Outport
  wires:
  bang-bang controller/1(out(+1/-1)) -> hydraulic lag/1
  hydraulic lag/1 -> braking pressure/1
  Integrator Limited/1 -> wheel speed/1  "wheel speed"
  Sum1/1 -> Gain/1
  error/1 -> bang-bang controller/1(error)
  braking pressure/1 -> force and torque/1  "braking torque"
  Gain/1 -> Integrator Limited/1
  tyre torque/1 -> Sum1/2
  force and torque/1 -> Sum1/1

== system SelfBalancingEV_V2/MODES/Bike ON//OFF ==
  u : Inport
  In2 : Inport  Port=2
  Compare To Zero : simulink/Logic and Bit Operations/Compare To Zero  relop===  OutDataTypeStr=boolean
  Off_speed : Constant  Value=0
  Switch : Switch  Criteria=u2 ~= 0  SaturateOnIntegerOverflow=off  InputSameDT=off
  Out1 : Outport
  wires:
  Compare To Zero/1 -> Switch/2
  Switch/1 -> Out1/1
  Off_speed/1 -> Switch/1
  In2/1 -> Switch/3
  u/1 -> Compare To Zero/1

== system SelfBalancingEV_V2/MODES/ECO_MODE ==
  u : Inport
  In2 : Inport  Port=2
  Compare To Constant Eco_mode : simulink/Logic and Bit Operations/Compare To Constant  relop===  const=2  OutDataTypeStr=boolean
  Eco_mode : Constant  Value=20
  Switch1 : Switch  Criteria=u2 ~= 0  SaturateOnIntegerOverflow=off  InputSameDT=off
  Out1 : Outport
  wires:
  Eco_mode/1 -> Switch1/1
  Compare To Constant Eco_mode/1 -> Switch1/2
  Switch1/1 -> Out1/1
  u/1 -> Compare To Constant Eco_mode/1
  In2/1 -> Switch1/3

== system SelfBalancingEV_V2/MODES/SPORTS_MODE ==
  u : Inport
  In2 : Inport  Port=2
  Compare To Constant Sports_mode : simulink/Logic and Bit Operations/Compare To Constant  relop===  const=4  OutDataTypeStr=boolean
  Sports_mode : Constant  Value=90
  Switch3 : Switch  Criteria=u2 ~= 0  SaturateOnIntegerOverflow=off  InputSameDT=off
  Out1 : Outport
  wires:
  Compare To Constant Sports_mode/1 -> Switch3/2
  Sports_mode/1 -> Switch3/1
  Switch3/1 -> Out1/1
  In2/1 -> Switch3/3
  u/1 -> Compare To Constant Sports_mode/1

== system SelfBalancingEV_V2/MODES/Self_Balance ==
  u : Inport
  Compare To Constant Self_balance : simulink/Logic and Bit Operations/Compare To Constant  relop===  const=1  OutDataTypeStr=boolean
  OFF : Constant  Value=0
  ON : Constant
  Switch4 : Switch  Criteria=u2 ~= 0  SaturateOnIntegerOverflow=off  InputSameDT=off
  Out1 : Outport
  wires:
  OFF/1 -> Switch4/3
  ON/1 -> Switch4/1
  Compare To Constant Self_balance/1 -> Switch4/2
  Switch4/1 -> Out1/1
  u/1 -> Compare To Constant Self_balance/1

== system SelfBalancingEV_V2/MODES/URBAN_MODE ==
  u : Inport
  In2 : Inport  Port=2
  Compare To Constant Urban_mode : simulink/Logic and Bit Operations/Compare To Constant  relop===  const=3  OutDataTypeStr=boolean
  Switch2 : Switch  Criteria=u2 ~= 0  SaturateOnIntegerOverflow=off  InputSameDT=off
  Urban_mode : Constant  Value=45
  Out1 : Outport
  wires:
  Switch2/1 -> Out1/1
  Compare To Constant Urban_mode/1 -> Switch2/2
  Urban_mode/1 -> Switch2/1
  u/1 -> Compare To Constant Urban_mode/1
  In2/1 -> Switch2/3

== system SelfBalancingEV_V2/MODES/WRONG_INPUT ==
  u : Inport
  Compare To Constant Wrong_input : simulink/Logic and Bit Operations/Compare To Constant  relop=>=  const=5  OutDataTypeStr=boolean
  NULL : Constant  Value=0
  Switch5 : Switch  Criteria=u2 ~= 0  SaturateOnIntegerOverflow=off  InputSameDT=off
  Out1 : Outport
  wires:
  Compare To Constant Wrong_input/1 -> Switch5/2
  NULL/1 -> Switch5/1
  u/1 -> Compare To Constant Wrong_input/1
  Switch5/1 -> Out1/1

== system SelfBalancingEV_V2/State of charge, current and voltage monitoring system/data acquisition system ==
  In1 : Inport
  Bus Selector1 : BusSelector  OutputSignals=SOC (%),Current (A),Voltage (V)
  <SOC (%)> : Outport
  <Current (A)> : Outport  Port=2
  <Voltage (V)> : Outport  Port=3
  wires:
  Bus Selector1/3 -> <Voltage (V)>/1  "<Voltage (V)>"
  Bus Selector1/2 -> <Current (A)>/1  "<Current (A)>"
  In1/1 -> Bus Selector1/1
  Bus Selector1/1 -> <SOC (%)>/1  "<SOC (%)>"

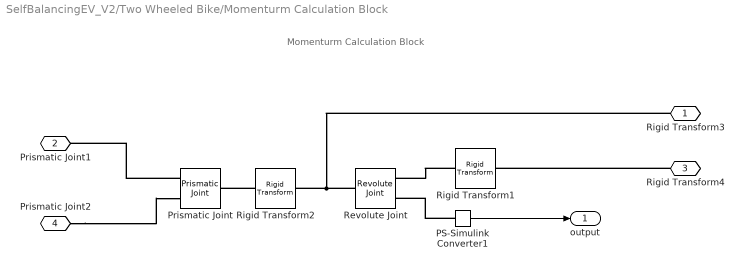
== system SelfBalancingEV_V2/Two Wheeled Bike/Momenturm Calculation Block ==
  note: Momenturm Calculation Block
  PS-Simulink Converter1 : nesl_utility/PS-Simulink Converter  PhysicalDomain=network_engine_domain  SubClassName=ps_output  LeftPortType=input  RightPortType=output  PseudoPeriodic=off  Frequencies=[]  VectorFormat=1-D array  Unit=rad  AffineConversion=off
  Prismatic Joint : sm_lib/Joints/Prismatic Joint  JointMode=Normal  SenseConstraintForce=off  SenseConstraintForceX=off  SenseConstraintForceY=off  SenseConstraintForceZ=off  SenseConstraintTorque=off  SenseConstraintTorqueX=off  SenseConstraintTorqueY=off  SenseConstraintTorqueZ=off  SenseTotalForce=off  SenseTotalForceX=off  SenseTotalForceY=off  SenseTotalForceZ=off  SenseTotalTorque=off  SenseTotalTorqueX=off  SenseTotalTorqueY=off  SenseTotalTorqueZ=off  CompositeWrenchDir=FollowerOnBase  CompositeWrenchFrame=BaseFrame  EquilibriumPosition=0  EquilibriumPositionUnits=m  SpringStiffness=0  SpringStiffnessUnits=N/m  DampingCoefficient=0  DampingCoefficientUnits=N/(m/s)  TorqueActuationMode=InputTorque  MotionActuationMode=ComputedMotion  SensePosition=off  SenseVelocity=off  SenseAcceleration=off  SenseTorqueForce=off  SenseLowerLimitTorqueForce=off  SenseUpperLimitTorqueForce=off  LowerLimitSpecify=off  LowerLimitBound=-1  LowerLimitBoundUnits=m  LowerLimitStiffness=1e6  LowerLimitStiffnessUnits=N/m  LowerLimitDamping=1e3  LowerLimitDampingUnits=N/(m/s)  LowerLimitTransitionRegionWidth=1e-4  LowerLimitTransitionRegionWidthUnits=m  UpperLimitSpecify=off  UpperLimitBound=1  UpperLimitBoundUnits=m  UpperLimitStiffness=1e6  UpperLimitStiffnessUnits=N/m  UpperLimitDamping=1e3  UpperLimitDampingUnits=N/(m/s)  UpperLimitTransitionRegionWidth=1e-4  UpperLimitTransitionRegionWidthUnits=m  PositionTargetSpecify=off  PositionTargetPriority=High  PositionTargetValue=0  PositionTargetValueUnits=m  VelocityTargetSpecify=off  VelocityTargetPriority=High  VelocityTargetValue=0  VelocityTargetValueUnits=m/s
  Revolute Joint : sm_lib/Joints/Revolute Joint  JointMode=Normal  SenseConstraintForce=off  SenseConstraintForceX=off  SenseConstraintForceY=off  SenseConstraintForceZ=off  SenseConstraintTorque=off  SenseConstraintTorqueX=off  SenseConstraintTorqueY=off  SenseConstraintTorqueZ=off  SenseTotalForce=off  SenseTotalForceX=off  SenseTotalForceY=off  SenseTotalForceZ=off  SenseTotalTorque=off  SenseTotalTorqueX=off  SenseTotalTorqueY=off  SenseTotalTorqueZ=off  CompositeWrenchDir=FollowerOnBase  CompositeWrenchFrame=BaseFrame  EquilibriumPosition=0  EquilibriumPositionUnits=deg  SpringStiffness=0  SpringStiffnessUnits=N*m/deg  DampingCoefficient=0.0003  DampingCoefficientUnits=N*m/(deg/s)  TorqueActuationMode=NoTorque  MotionActuationMode=ComputedMotion  SensePosition=on  SenseVelocity=off  SenseAcceleration=off  SenseTorqueForce=off  SenseLowerLimitTorqueForce=off  SenseUpperLimitTorqueForce=off  LowerLimitSpecify=off  LowerLimitBound=-90  LowerLimitBoundUnits=deg  LowerLimitStiffness=1e4  LowerLimitStiffnessUnits=N*m/deg  LowerLimitDamping=10  LowerLimitDampingUnits=N*m/(deg/s)  LowerLimitTransitionRegionWidth=0.1  LowerLimitTransitionRegionWidthUnits=deg  UpperLimitSpecify=off  UpperLimitBound=90  UpperLimitBoundUnits=deg  UpperLimitStiffness=1e4  UpperLimitStiffnessUnits=N*m/deg  UpperLimitDamping=10  UpperLimitDampingUnits=N*m/(deg/s)  UpperLimitTransitionRegionWidth=0.1  UpperLimitTransitionRegionWidthUnits=deg  PositionTargetSpecify=off  PositionTargetPriority=High  PositionTargetValue=0  PositionTargetValueUnits=deg  VelocityTargetSpecify=off  VelocityTargetPriority=High  VelocityTargetValue=0  VelocityTargetValueUnits=deg/s
  Rigid Transform1 : sm_lib/Frames and Transforms/Rigid Transform  TranslationMethod=None  TranslationStandardOffset=0  TranslationLengthUnit=m  TranslationStandardAxis=+Z  TranslationCartesianOffset=[0 0 0]  TranslationROffset=0  TranslationROffsetUnits=m  TranslationZOffset=0  TranslationZOffsetUnits=m  TranslationThetaOffset=0  TranslationThetaOffsetUnits=deg  RotationMethod=RotationSequence  RotationAngleUnits=deg  RotationStandardAxis=+Z  RotationAngle=0.0  RotationArbitraryAxis=[0 0 1]  FollAlignAxisA=+X  BaseAlignAxisA=+Y  FollAlignAxisB=+Y  BaseAlignAxisB=+Z  RotationSequenceAxes=FollowerAxes  RotationSequence=YXZ  RotationSequenceAngles=[90 180 0]  RotationSequenceAnglesUnits=deg  RotationMatrix=[1 0 0; 0 1 0; 0 0 1]
  Rigid Transform2 : sm_lib/Frames and Transforms/Rigid Transform  TranslationMethod=None  TranslationStandardOffset=0  TranslationLengthUnit=m  TranslationStandardAxis=+Z  TranslationCartesianOffset=[0 0 0]  TranslationROffset=0  TranslationROffsetUnits=m  TranslationZOffset=0  TranslationZOffsetUnits=m  TranslationThetaOffset=0  TranslationThetaOffsetUnits=deg  RotationMethod=RotationSequence  RotationAngleUnits=deg  RotationStandardAxis=+X  RotationAngle=90  RotationArbitraryAxis=[0 0 1]  FollAlignAxisA=+X  BaseAlignAxisA=+Y  FollAlignAxisB=+Y  BaseAlignAxisB=+Z  RotationSequenceAxes=FollowerAxes  RotationSequence=XYX  RotationSequenceAngles=[90 180 0]  RotationSequenceAnglesUnits=deg  RotationMatrix=[1 0 0; 0 1 0; 0 0 1]
  Rigid Transform3 : PMIOPort  Side=Right
  Prismatic Joint1 : PMIOPort  Port=2  Side=Left
  Rigid Transform4 : PMIOPort  Port=3  Side=Right
  Prismatic Joint2 : PMIOPort  Port=4  Side=Left
  output : Outport
  wires:
  PS-Simulink Converter1/1 -> output/1
  connections:
  Rigid Transform2/LConn1 -- Prismatic Joint/RConn1
  Revolute Joint/LConn1 -- Rigid Transform3/RConn1 -- Rigid Transform2/RConn1
  Rigid Transform4/RConn1 -- Rigid Transform1/RConn1
  Prismatic Joint2/RConn1 -- Prismatic Joint/LConn2
  PS-Simulink Converter1/LConn1 -- Revolute Joint/RConn2
  Rigid Transform1/LConn1 -- Revolute Joint/RConn1
  Prismatic Joint/LConn1 -- Prismatic Joint1/RConn1

== system SelfBalancingEV_V2/Two Wheeled Bike/Physical Block ==
  note: Physical Block
  cart : Subsystem
  chassis : Subsystem
  Conn1 : PMIOPort  Side=Left
  Conn2 : PMIOPort  Port=2  Side=Left
  connections:
  cart/LConn1 -- Conn1/RConn1
  chassis/LConn1 -- Conn2/RConn1

== system SelfBalancingEV_V2/Two Wheeled Bike/World Frame ==
  Mechanism Configuration : sm_lib/Utilities/Mechanism Configuration  UniformGravity=Constant  GravityVector=[-9.80665 0 0]  GravityVectorUnits=m/s^2  GravityUnits=m/s^2  LinearizationDelta=0.001  JointModeTransitionNonlinearIterations=2
  Solver Configuration : nesl_utility/Solver Configuration  PhysicalDomain=network_engine_domain  SubClassName=solver  LeftPortType=input  RightPortType=generic  Tones=[]  Harmonics=[]  SimulateNoise=off  Profile=off  UseLocalSampling=off  EnableSwitchedLinearOptims=on  FrequencyDomain=off  UseCCode=off  RelTol=0.001  AbsTol=1e-06  MinStep=1e-09  ToWorkspace=off  RevertToSquareIcSolve=off  NumHomotopyIterations=100  PhasorMode=off  PhasorModeNumHarmonics=1  IndexReductionMethod=DerivativeReplacement  DoDC=off  ResidualTolerance=1e-09  UseLocalSolver=off  LocalSolverChoice=NE_BACKWARD_EULER_ADVANCER  LocalSolverSampleTime=0.001  DoFixedCost=off  MaxNonlinIter=3  MaxModeIter=2  ComputeImpulses=off  ImpulseIterations=2  LinearAlgebra=Sparse  LinearAlgebraNumThread=0  EquationFormulation=NE_TIME_EF  DelaysMemoryBudget=1024  AutomaticFiltering=on  FilteringTimeConstant=0.001  PartitionStorageMethod=AS_NEEDED  PartitionMemoryBudget=1024  PartitionMethod=FAST
  World Frame : sm_lib/Frames and Transforms/World Frame
  a : PMIOPort  Side=Right
  connections:
  World Frame/RConn1 -- a/RConn1 -- Solver Configuration/RConn1 -- Mechanism Configuration/RConn1

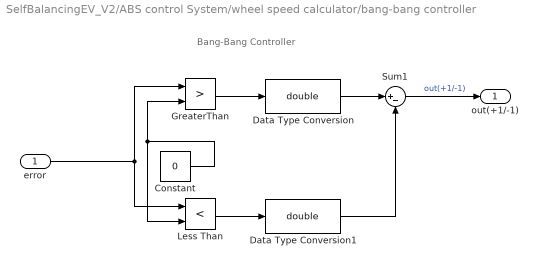
== system SelfBalancingEV_V2/ABS control System/wheel speed calculator/bang-bang controller ==
  note: Bang-Bang Controller
  error : Inport
  Constant : Constant  Value=0
  Data Type Conversion : DataTypeConversion  OutDataTypeStr=double  SaturateOnIntegerOverflow=off
  Data Type Conversion1 : DataTypeConversion  OutDataTypeStr=double  SaturateOnIntegerOverflow=off
  GreaterThan : RelationalOperator  Operator=>  OutDataTypeStr=boolean  RndMeth=Simplest  InputSameDT=off
  Less Than : RelationalOperator  Operator=<  OutDataTypeStr=boolean  RndMeth=Simplest  InputSameDT=off
  Sum1 : Sum  Inputs=|+-
  out(+1/-1) : Outport
  wires:
  Constant/1 -> GreaterThan/2, Less Than/2
  Data Type Conversion/1 -> Sum1/1
  GreaterThan/1 -> Data Type Conversion/1
  Less Than/1 -> Data Type Conversion1/1
  error/1 -> GreaterThan/1, Less Than/1
  Data Type Conversion1/1 -> Sum1/2
  Sum1/1 -> out(+1/-1)/1  "out(+1/-1)"

== system SelfBalancingEV_V2/Two Wheeled Bike/Physical Block/cart ==
  Rigid Transform1 : sm_lib/Frames and Transforms/Rigid Transform  TranslationMethod=StandardAxis  TranslationStandardOffset=10  TranslationLengthUnit=cm  TranslationStandardAxis=+Z  TranslationCartesianOffset=[0 0 0]  TranslationROffset=0  TranslationROffsetUnits=m  TranslationZOffset=0  TranslationZOffsetUnits=m  TranslationThetaOffset=0  TranslationThetaOffsetUnits=deg  RotationMethod=None  RotationAngleUnits=deg  RotationStandardAxis=+Z  RotationAngle=0.0  RotationArbitraryAxis=[0 0 1]  FollAlignAxisA=+X  BaseAlignAxisA=+Y  FollAlignAxisB=+Y  BaseAlignAxisB=+Z  RotationSequenceAxes=FollowerAxes  RotationSequence=XYX  RotationSequenceAngles=[0 0 0]  RotationSequenceAnglesUnits=deg  RotationMatrix=[1 0 0; 0 1 0; 0 0 1]
  Rigid Transform2 : sm_lib/Frames and Transforms/Rigid Transform  TranslationMethod=StandardAxis  TranslationStandardOffset=10  TranslationLengthUnit=cm  TranslationStandardAxis=-Z  TranslationCartesianOffset=[0 0 0]  TranslationROffset=0  TranslationROffsetUnits=m  TranslationZOffset=0  TranslationZOffsetUnits=m  TranslationThetaOffset=0  TranslationThetaOffsetUnits=deg  RotationMethod=None  RotationAngleUnits=deg  RotationStandardAxis=+Z  RotationAngle=0.0  RotationArbitraryAxis=[0 0 1]  FollAlignAxisA=+X  BaseAlignAxisA=+Y  FollAlignAxisB=+Y  BaseAlignAxisB=+Z  RotationSequenceAxes=FollowerAxes  RotationSequence=XYX  RotationSequenceAngles=[0 0 0]  RotationSequenceAnglesUnits=deg  RotationMatrix=[1 0 0; 0 1 0; 0 0 1]
  "left wheel " : Subsystem
  "right wheel " : Subsystem
  "shaft " : sm_lib/Body Elements/Brick Solid  GraphicAmbientColor=[0.15 0.15 0.15 1.0]  BasedOnType=Mass  BrickDimensions=[1 1 20]  BrickDimensionUnits=cm  CenterOfMass=[0 0 0]  CenterOfMassUnits=m  GraphicDiffuseColor=[0.5 0.5 0.5]  Density=1000  DensityUnits=kg/m^3  DoExposeReferenceFrame=on  GraphicEmissiveColor=[0.0 0.0 0.0 1.0]  ExportEntireGeometry=off  SerializedFrames=<Frames/>  MarkerShape=Sphere  MarkerSize=10  GraphicType=FromGeometry  InertiaType=CalculateFromGeometry  Mass=100  MassUnits=g  MomentsOfInertia=[1 1 1]  MomentsOfInertiaUnits=kg*m^2  GraphicOpacity=1.0  ProductsOfInertia=[0 0 0]  ProductsOfInertiaUnits=kg*m^2  GraphicShininess=75  GraphicSpecularColor=[0.5 0.5 0.5 1.0]  GraphicVisPropType=SimpleVisualProperties
  Conn1 : PMIOPort  Side=Left
  connections:
  "left wheel "/LConn1 -- Rigid Transform2/RConn1
  "right wheel "/LConn1 -- Rigid Transform1/RConn1
  Rigid Transform1/LConn1 -- Rigid Transform2/LConn1 -- Conn1/RConn1 -- "shaft "/RConn1

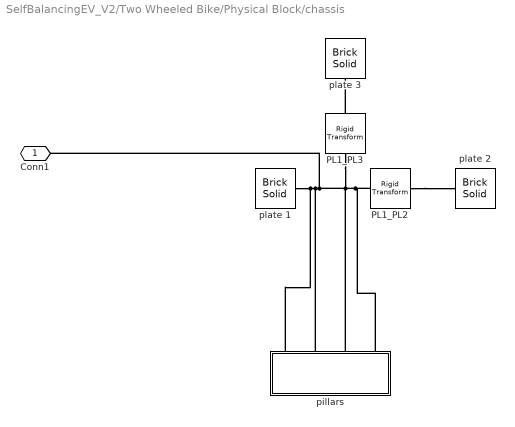
== system SelfBalancingEV_V2/Two Wheeled Bike/Physical Block/chassis ==
  "PL1_PL2 " : sm_lib/Frames and Transforms/Rigid Transform  TranslationMethod=StandardAxis  TranslationStandardOffset=10  TranslationLengthUnit=cm  TranslationStandardAxis=+Z  TranslationCartesianOffset=[0 0 0]  TranslationROffset=0  TranslationROffsetUnits=m  TranslationZOffset=0  TranslationZOffsetUnits=m  TranslationThetaOffset=0  TranslationThetaOffsetUnits=deg  RotationMethod=None  RotationAngleUnits=deg  RotationStandardAxis=+Z  RotationAngle=0.0  RotationArbitraryAxis=[0 0 1]  FollAlignAxisA=+X  BaseAlignAxisA=+Y  FollAlignAxisB=+Y  BaseAlignAxisB=+Z  RotationSequenceAxes=FollowerAxes  RotationSequence=XYX  RotationSequenceAngles=[0 0 0]  RotationSequenceAnglesUnits=deg  RotationMatrix=[1 0 0; 0 1 0; 0 0 1]
  "PL1_PL3 " : sm_lib/Frames and Transforms/Rigid Transform  TranslationMethod=StandardAxis  TranslationStandardOffset=25  TranslationLengthUnit=cm  TranslationStandardAxis=+Z  TranslationCartesianOffset=[0 0 0]  TranslationROffset=0  TranslationROffsetUnits=m  TranslationZOffset=0  TranslationZOffsetUnits=m  TranslationThetaOffset=0  TranslationThetaOffsetUnits=deg  RotationMethod=None  RotationAngleUnits=deg  RotationStandardAxis=+Z  RotationAngle=0.0  RotationArbitraryAxis=[0 0 1]  FollAlignAxisA=+X  BaseAlignAxisA=+Y  FollAlignAxisB=+Y  BaseAlignAxisB=+Z  RotationSequenceAxes=FollowerAxes  RotationSequence=XYX  RotationSequenceAngles=[0 0 0]  RotationSequenceAnglesUnits=deg  RotationMatrix=[1 0 0; 0 1 0; 0 0 1]
  "pillars " : Subsystem
  plate 1 : sm_lib/Body Elements/Brick Solid  GraphicAmbientColor=[0.15 0.15 0.15 1.0]  BasedOnType=Mass  BrickDimensions=[18 8 0.3]  BrickDimensionUnits=cm  CenterOfMass=[0 0 0]  CenterOfMassUnits=m  GraphicDiffuseColor=[1.0 0.4 0.4]  Density=1000  DensityUnits=kg/m^3  DoExposeReferenceFrame=on  GraphicEmissiveColor=[0.0 0.0 0.0 1.0]  ExportEntireGeometry=off  SerializedFrames=<Frames/>  MarkerShape=Sphere  MarkerSize=10  GraphicType=FromGeometry  InertiaType=CalculateFromGeometry  Mass=1/4  MassUnits=kg  MomentsOfInertia=[1 1 1]  MomentsOfInertiaUnits=kg*m^2  GraphicOpacity=0.6  ProductsOfInertia=[0 0 0]  ProductsOfInertiaUnits=kg*m^2  GraphicShininess=75  GraphicSpecularColor=[0.5 0.5 0.5 1.0]  GraphicVisPropType=SimpleVisualProperties
  "plate 2 " : sm_lib/Body Elements/Brick Solid  GraphicAmbientColor=[0.15 0.15 0.15 1.0]  BasedOnType=Mass  BrickDimensions=[18 8 0.3]  BrickDimensionUnits=cm  CenterOfMass=[0 0 0]  CenterOfMassUnits=m  GraphicDiffuseColor=[1.0 0.4 0.4]  Density=1000  DensityUnits=kg/m^3  DoExposeReferenceFrame=on  GraphicEmissiveColor=[0.0 0.0 0.0 1.0]  ExportEntireGeometry=off  SerializedFrames=<Frames/>  MarkerShape=Sphere  MarkerSize=10  GraphicType=FromGeometry  InertiaType=CalculateFromGeometry  Mass=1/4  MassUnits=kg  MomentsOfInertia=[1 1 1]  MomentsOfInertiaUnits=kg*m^2  GraphicOpacity=0.6  ProductsOfInertia=[0 0 0]  ProductsOfInertiaUnits=kg*m^2  GraphicShininess=75  GraphicSpecularColor=[0.5 0.5 0.5 1.0]  GraphicVisPropType=SimpleVisualProperties
  plate 3 : sm_lib/Body Elements/Brick Solid  GraphicAmbientColor=[0.15 0.15 0.15 1.0]  BasedOnType=Mass  BrickDimensions=[18 8 0.3]  BrickDimensionUnits=cm  CenterOfMass=[0 0 0]  CenterOfMassUnits=m  GraphicDiffuseColor=[1.0 0.4 0.4]  Density=1000  DensityUnits=kg/m^3  DoExposeReferenceFrame=on  GraphicEmissiveColor=[0.0 0.0 0.0 1.0]  ExportEntireGeometry=off  SerializedFrames=<Frames/>  MarkerShape=Sphere  MarkerSize=10  GraphicType=FromGeometry  InertiaType=CalculateFromGeometry  Mass=1/4  MassUnits=kg  MomentsOfInertia=[1 1 1]  MomentsOfInertiaUnits=kg*m^2  GraphicOpacity=0.6  ProductsOfInertia=[0 0 0]  ProductsOfInertiaUnits=kg*m^2  GraphicShininess=75  GraphicSpecularColor=[0.5 0.5 0.5 1.0]  GraphicVisPropType=SimpleVisualProperties
  Conn1 : PMIOPort  Side=Left
  connections:
  "pillars "/LConn3 -- Conn1/RConn1 -- "pillars "/LConn2 -- "pillars "/LConn1 -- plate 1/RConn1 -- "pillars "/LConn4 -- "PL1_PL2 "/LConn1 -- "PL1_PL3 "/LConn1
  "PL1_PL3 "/RConn1 -- plate 3/RConn1
  "PL1_PL2 "/RConn1 -- "plate 2 "/RConn1

== system SelfBalancingEV_V2/Two Wheeled Bike/Physical Block/cart/left wheel  ==
  "left wheel tyre " : sm_lib/Body Elements/Cylindrical Solid  GraphicAmbientColor=[0.15 0.15 0.15 1.0]  BasedOnType=Mass  CenterOfMass=[0 0 0]  CenterOfMassUnits=m  GraphicDiffuseColor=[0.0 0.0 0.0]  CylinderLength=12.5  CylinderLengthUnits=mm  CylinderRadius=32.5  CylinderRadiusUnits=mm  Density=1000  DensityUnits=kg/m^3  DoExposeReferenceFrame=on  GraphicEmissiveColor=[0.0 0.0 0.0 1.0]  ExportEntireGeometry=off  SerializedFrames=<Frames/>  MarkerShape=Sphere  MarkerSize=10  GraphicType=FromGeometry  InertiaType=PointMass  Mass=2  MassUnits=g  MomentsOfInertia=[1 1 1]  MomentsOfInertiaUnits=kg*m^2  GraphicOpacity=1.0  ProductsOfInertia=[0 0 0]  ProductsOfInertiaUnits=kg*m^2  GraphicShininess=75  GraphicSpecularColor=[0.5 0.5 0.5 1.0]  GraphicVisPropType=SimpleVisualProperties
  left wheel wheel body : sm_lib/Body Elements/Cylindrical Solid  GraphicAmbientColor=[0.15 0.15 0.15 1.0]  BasedOnType=Density  CenterOfMass=[0 0 0]  CenterOfMassUnits=m  GraphicDiffuseColor=[1.0 1.0 0.2]  CylinderLength=12.7  CylinderLengthUnits=mm  CylinderRadius=30  CylinderRadiusUnits=mm  Density=2  DensityUnits=g  DoExposeReferenceFrame=on  GraphicEmissiveColor=[0.0 0.0 0.0 1.0]  ExportEntireGeometry=off  SerializedFrames=<Frames/>  MarkerShape=Sphere  MarkerSize=10  GraphicType=FromGeometry  InertiaType=PointMass  Mass=48  MassUnits=g  MomentsOfInertia=[1 1 1]  MomentsOfInertiaUnits=kg*m^2  GraphicOpacity=1.0  ProductsOfInertia=[0 0 0]  ProductsOfInertiaUnits=kg*m^2  GraphicShininess=75  GraphicSpecularColor=[0.5 0.5 0.5 1.0]  GraphicVisPropType=SimpleVisualProperties
  Conn1 : PMIOPort  Side=Left
  connections:
  "left wheel tyre "/RConn1 -- left wheel wheel body/RConn1 -- Conn1/RConn1

== system SelfBalancingEV_V2/Two Wheeled Bike/Physical Block/cart/right wheel  ==
  "left wheel tyre " : sm_lib/Body Elements/Cylindrical Solid  GraphicAmbientColor=[0.15 0.15 0.15 1.0]  BasedOnType=Mass  CenterOfMass=[0 0 0]  CenterOfMassUnits=m  GraphicDiffuseColor=[0.0 0.0 0.0]  CylinderLength=12.5  CylinderLengthUnits=mm  CylinderRadius=32.5  CylinderRadiusUnits=mm  Density=1000  DensityUnits=kg/m^3  DoExposeReferenceFrame=on  GraphicEmissiveColor=[0.0 0.0 0.0 1.0]  ExportEntireGeometry=off  SerializedFrames=<Frames/>  MarkerShape=Sphere  MarkerSize=10  GraphicType=FromGeometry  InertiaType=PointMass  Mass=2  MassUnits=g  MomentsOfInertia=[1 1 1]  MomentsOfInertiaUnits=kg*m^2  GraphicOpacity=1.0  ProductsOfInertia=[0 0 0]  ProductsOfInertiaUnits=kg*m^2  GraphicShininess=75  GraphicSpecularColor=[0.5 0.5 0.5 1.0]  GraphicVisPropType=SimpleVisualProperties
  left wheel wheel body : sm_lib/Body Elements/Cylindrical Solid  GraphicAmbientColor=[0.15 0.15 0.15 1.0]  BasedOnType=Density  CenterOfMass=[0 0 0]  CenterOfMassUnits=m  GraphicDiffuseColor=[1.0 1.0 0.2]  CylinderLength=12.7  CylinderLengthUnits=mm  CylinderRadius=30  CylinderRadiusUnits=mm  Density=2  DensityUnits=g  DoExposeReferenceFrame=on  GraphicEmissiveColor=[0.0 0.0 0.0 1.0]  ExportEntireGeometry=off  SerializedFrames=<Frames/>  MarkerShape=Sphere  MarkerSize=10  GraphicType=FromGeometry  InertiaType=PointMass  Mass=48  MassUnits=g  MomentsOfInertia=[1 1 1]  MomentsOfInertiaUnits=kg*m^2  GraphicOpacity=1.0  ProductsOfInertia=[0 0 0]  ProductsOfInertiaUnits=kg*m^2  GraphicShininess=75  GraphicSpecularColor=[0.5 0.5 0.5 1.0]  GraphicVisPropType=SimpleVisualProperties
  Conn1 : PMIOPort  Side=Left
  connections:
  "left wheel tyre "/RConn1 -- left wheel wheel body/RConn1 -- Conn1/RConn1
